simulink subsystem "Actuator_to_Engineering"  (R2025a)
settings: Solver=VariableStepAuto  StartTime=0.0  StopTime=10.0  RelTol=1e-3
undefined symbols (not defined in the file or in its folder): vehicle
settings Model: Creator=gurt1  LastModifiedBy=17036

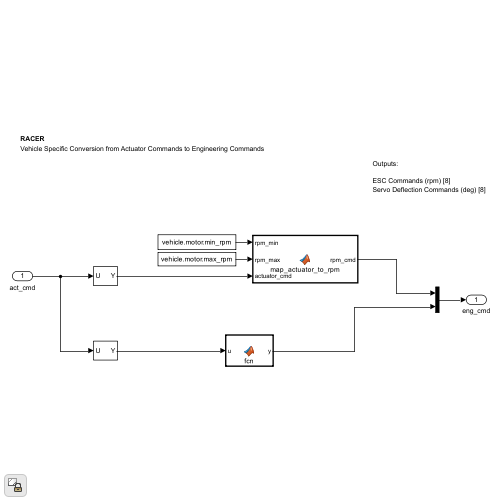
[thumbnail: Simulink's stored preview of the top-level diagram]
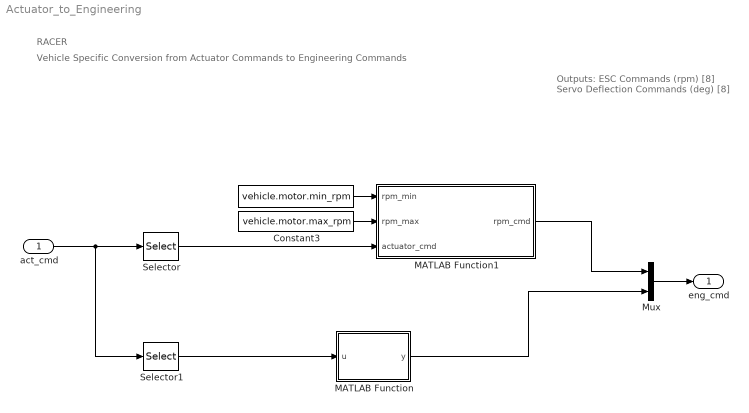
== system Actuator_to_Engineering ==
  note: Outputs:
      |
      | ESC Commands (rpm) [8]
      | Servo Deflection Commands (deg) [8]
  note: RACER
  note: Vehicle Specific Conversion from Actuator Commands to Engineering Commands
  act_cmd : Inport
  " " : Constant  Value=vehicle.motor.min_rpm
  Constant3 : Constant  Value=vehicle.motor.max_rpm
  MATLAB Function : MATLAB Function  TreatAsAtomicUnit=on
  MATLAB Function1 : MATLAB Function  TreatAsAtomicUnit=on
  Mux : Mux  Inputs=2
  Selector : Selector  InputPortWidth=16  IndexOptions=Index vector (dialog)  Indices=[1:8]  OutputSizes=1
  Selector1 : Selector  InputPortWidth=16  IndexOptions=Index vector (dialog)  Indices=[9:16]  OutputSizes=1
  eng_cmd : Outport
  wires:
  act_cmd/1 -> Selector/1, Selector1/1
  " "/1 -> MATLAB Function1/1(rpm_min)
  Constant3/1 -> MATLAB Function1/2(rpm_max)
  Selector/1 -> MATLAB Function1/3(actuator_cmd)
  Mux/1 -> eng_cmd/1
  MATLAB Function1/1(rpm_cmd) -> Mux/1
  Selector1/1 -> MATLAB Function/1(u)
  MATLAB Function/1(y) -> Mux/2

== matlab function Actuator_to_Engineering/MATLAB Function ==
  data: u input; y output
function y = fcn(u)

y = u;

== matlab function Actuator_to_Engineering/MATLAB Function1 ==
  data: rpm_min input; rpm_cmd output; rpm_max input; actuator_cmd input
function rpm_cmd = map_actuator_to_rpm(rpm_min, rpm_max, actuator_cmd)

rpm_cmd = map_actuator_to_rpm(rpm_min, rpm_max, actuator_cmd);
